simulink model "mission_server_leader_follower_qbot2_qbot2"  (Simulink 8.3)
settings: Solver=FixedStepDiscrete  StartTime=0.0  StopTime=inf  FixedStep=0.002  RelTol=1e-3
libraries: quarc_library x5, Orientation_Library x4
settings Model: Creator=glai  LastModifiedBy=user  SimulationMode=external  ExtModeTrigDuration=5000
settings SolverCC: PositivePriorityOrder=on
settings DataIOCC: SignalLoggingSaveFormat=Dataset
settings OptimizationCC: ExpressionDepthLimit=2147483647
settings RTWCC: SystemTargetFile=quarc_win64.tlc  TemplateMakefile=quarc_default_tmf  Description=QUARC Win64 Target  ProcessScript=quarc_win64_make_rtw_hook
settings STFCustomTargetCC: TargetPreCompLibLocation=C:\PROGRA~3\QUARC\lib\2014a\win64\release  CodeReplacementLibrary=C89/C90 (ANSI)  ConcurrentExecutionCompliant=on  GeneratePreprocessorConditionals=Disable all  CombineOutputUpdateFcns=on  CPPClassGenCompliant=on  GRTInterface=off  SystemTargetFile=quarc_win64.tlc
settings GRTTargetCC: TargetPreCompLibLocation=C:\PROGRA~3\QUARC\lib\2014a\win64\release  CodeReplacementLibrary=C89/C90 (ANSI)  ParMdlRefBuildCompliant=off  CompOptLevelCompliant=off  CombineOutputUpdateFcns=on  MatFileLogging=off  GRTInterface=off  ExtMode=on  ExtModeMexFile=quarc_comm  ExtModeMexArgs='-w -d %d -uri %u','shmem://%m:1?timeout=10'

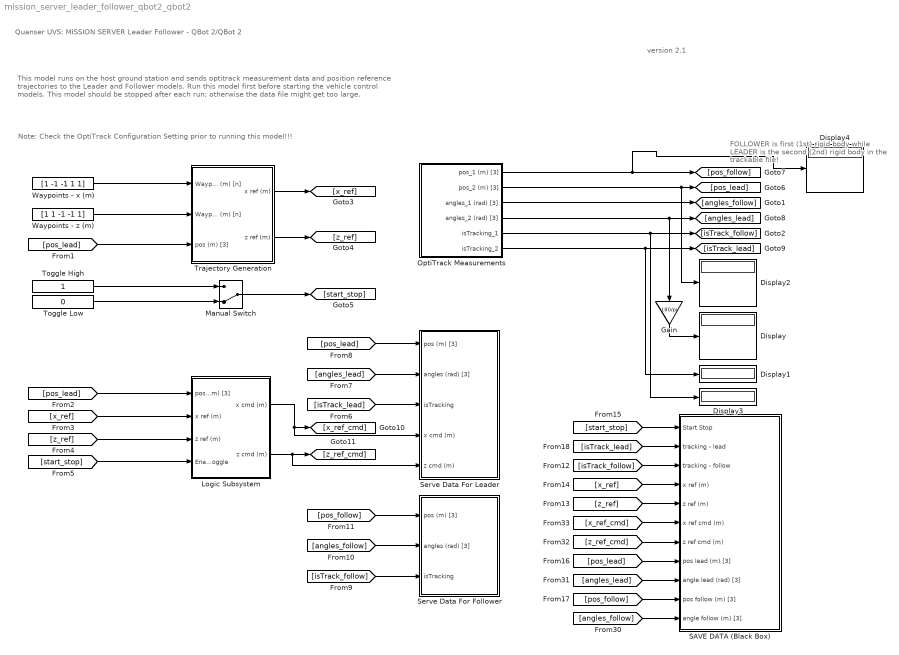
== system mission_server_leader_follower_qbot2_qbot2 ==
  note: FOLLOWER is first (1st) rigid body while
      | LEADER is the second (2nd) rigid body
      | in the trackable file!
  note: Note: Check the OptiTrack Configuration Setting prior to running this model!!!
  note: Quanser UVS: MISSION SERVER Leader Follower - QBot 2/QBot 2
  note: This model runs on the host ground station and sends
      | optitrack measurement data and position reference trajectories to the Leader and Follower models.
      | Run this model first before starting the vehicle control models.
      | This model should be stopped after each run; otherwise the data file might get too large.
  note: version 2.1
  Display{,1..4} (5 alike) : Display
      settings: Decimation=100
  Gain : Gain  Gain=180/pi
  Logic Subsystem : Subsystem
  Manual Switch : ManualSwitch  CurrentSetting=0
  OptiTrack Measurements : Subsystem
  SAVE DATA (Black Box) : Subsystem
  Serve Data For Follower : Subsystem
  Serve Data For Leader : Subsystem
  Toggle High : Constant
  Toggle Low : Constant  Value=0
  Trajectory Generation : Subsystem
  Waypoints - x (m) : Constant  Value=[1 -1 -1 1 1]
  Waypoints - z (m) : Constant  Value=[1 1 -1 -1 1]
  wires:
  Trajectory Generation/2(z ref (m)) -> [z_ref]
  Trajectory Generation/1(x ref (m)) -> [x_ref]
  [pos_lead] -> Logic Subsystem/1(pos (m) [3])
  [x_ref] -> Logic Subsystem/2(x ref (m))
  [start_stop] -> Logic Subsystem/4(Enable Toggle)
  [z_ref] -> Logic Subsystem/3(z ref (m))
  Logic Subsystem/1(x cmd (m)) -> [x_ref_cmd], Serve Data For Leader/4(x cmd (m))
  Logic Subsystem/2(z cmd (m)) -> [z_ref_cmd], Serve Data For Leader/5(z cmd (m))
  [angles_lead] -> Serve Data For Leader/2(angles (rad) [3])
  [isTrack_lead] -> Serve Data For Leader/3(isTracking)
  [pos_lead] -> Serve Data For Leader/1(pos (m) [3])
  Toggle High/1 -> Manual Switch/1
  Toggle Low/1 -> Manual Switch/2
  Manual Switch/1 -> [start_stop]
  Gain/1 -> Display/1
  OptiTrack Measurements/6(isTracking_2) -> Display1/1, [isTrack_lead]
  OptiTrack Measurements/5(isTracking_1) -> Display3/1, [isTrack_follow]
  OptiTrack Measurements/2(pos_2 (m) [3]) -> Display2/1, [pos_lead]
  OptiTrack Measurements/1(pos_1 (m) [3]) -> Display4/1, [pos_follow]
  OptiTrack Measurements/4(angles_2 (rad) [3]) -> Gain/1, [angles_lead]
  OptiTrack Measurements/3(angles_1 (rad) [3]) -> [angles_follow]
  [pos_follow] -> Serve Data For Follower/1(pos (m) [3])
  [angles_follow] -> Serve Data For Follower/2(angles (rad) [3])
  [isTrack_follow] -> Serve Data For Follower/3(isTracking)
  [z_ref] -> SAVE DATA (Black Box)/5(z ref (m))
  [start_stop] -> SAVE DATA (Black Box)/1(Start Stop)
  [x_ref] -> SAVE DATA (Black Box)/4(x ref (m))
  [pos_lead] -> SAVE DATA (Black Box)/8(pos lead (m) [3])
  [pos_follow] -> SAVE DATA (Black Box)/10(pos follow (m) [3])
  [angles_follow] -> SAVE DATA (Black Box)/11(angle follow (m) [3])
  [angles_lead] -> SAVE DATA (Black Box)/9(angle lead (rad) [3])
  [isTrack_follow] -> SAVE DATA (Black Box)/3(tracking - follow)
  [isTrack_lead] -> SAVE DATA (Black Box)/2(tracking - lead)
  [z_ref_cmd] -> SAVE DATA (Black Box)/7(z ref cmd (m))
  [x_ref_cmd] -> SAVE DATA (Black Box)/6(x ref cmd (m))
  Waypoints - z (m)/1 -> Trajectory Generation/2(Waypoint Z (m) [n])
  Waypoints - x (m)/1 -> Trajectory Generation/1(Waypoint X (m) [n])
  [pos_lead] -> Trajectory Generation/3(pos (m) [3])

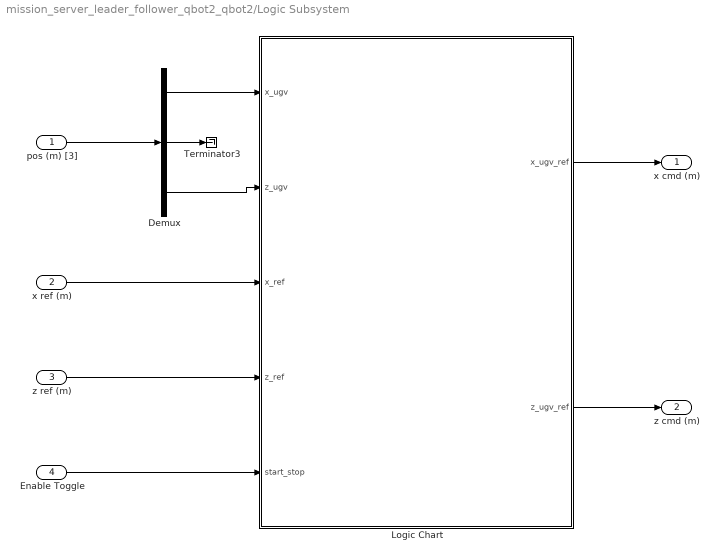
== system mission_server_leader_follower_qbot2_qbot2/Logic Subsystem ==
  pos (m) [3] : Inport
  x ref (m) : Inport  Port=2
  z ref (m) : Inport  Port=3
  Enable Toggle : Inport  Port=4
  Demux : Demux  Outputs=3
  Logic Chart : Stateflow chart  TreatAsAtomicUnit=on
  Terminator3 : Terminator
  x cmd (m) : Outport
  z cmd (m) : Outport  Port=2
  wires:
  pos (m) [3]/1 -> Demux/1
  Demux/2 -> Terminator3/1
  Demux/1 -> Logic Chart/1(x_ugv)
  Demux/3 -> Logic Chart/2(z_ugv)
  z ref (m)/1 -> Logic Chart/4(z_ref)
  Enable Toggle/1 -> Logic Chart/5(start_stop)
  x ref (m)/1 -> Logic Chart/3(x_ref)
  Logic Chart/1(x_ugv_ref) -> x cmd (m)/1
  Logic Chart/2(z_ugv_ref) -> z cmd (m)/1

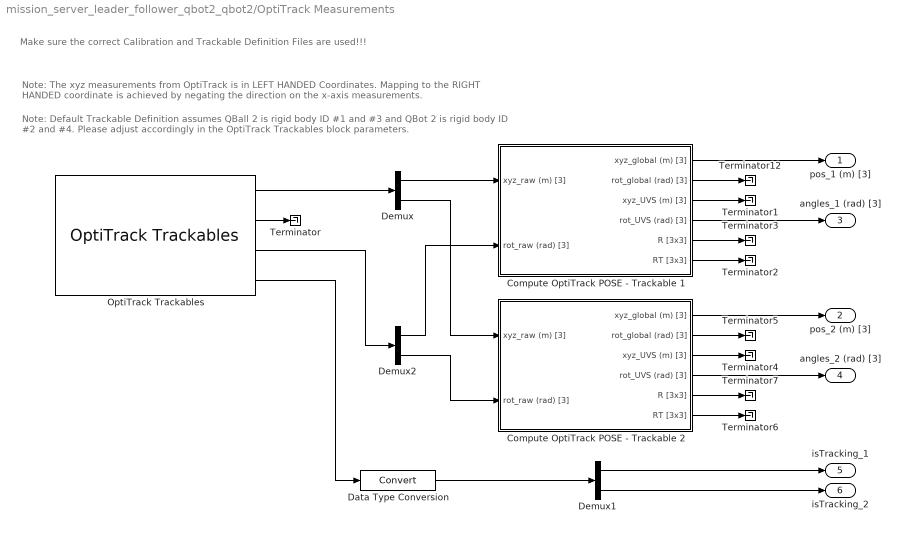
== system mission_server_leader_follower_qbot2_qbot2/OptiTrack Measurements ==
  note: Note: The xyz measurements from OptiTrack is in LEFT HANDED Coordinates.
      |
      | Mapping to the RIGHT HANDED coordinate is achieved by negating the direction on the x-axis measurements.
  note: Make sure the correct Calibration and Trackable Definition Files are used!!!
  note: Note: Default Trackable Definition assumes QBall 2 is rigid body ID #1 and #3 and QBot 2 is rigid body ID #2 and #4.
      | Please adjust accordingly in the OptiTrack Trackables block parameters.
  "Compute OptiTrack POSE - Trackable 1 " : Subsystem
  Compute OptiTrack POSE - Trackable 2 : Subsystem
  Data Type Conversion : DataTypeConversion
  Demux : Demux  Outputs=2
  Demux1 : Demux  Outputs=2
  Demux2 : Demux  Outputs=2
  OptiTrack Trackables : quarc_library/Devices/Third-Party/NaturalPoint/OptiTrack/OptiTrack Trackables  calibration_file=C:\Users\user\Desktop\final\Calibration Very High Quality Exceptional (MeanErr 0.001 mm) 2017-05-16 6.48pm.cal  rigid_body_file=C:\Users\user\Desktop\final\RigidBodies 2017-05-26 5.36pm_qbotx2.tra  rigid_body_ids=[1 2]  sample_time=qc_get_step_size
  Terminator{,1..7,12} (9 alike) : Terminator
  pos_1 (m) [3] : Outport
  pos_2 (m) [3] : Outport  Port=2
  angles_1 (rad) [3] : Outport  Port=3
  angles_2 (rad) [3] : Outport  Port=4
  isTracking_1 : Outport  Port=5
  isTracking_2 : Outport  Port=6
  wires:
  OptiTrack Trackables/1 -> Demux/1
  OptiTrack Trackables/2 -> Terminator/1
  OptiTrack Trackables/4 -> Data Type Conversion/1
  Data Type Conversion/1 -> Demux1/1
  Demux1/1 -> isTracking_1/1
  Demux1/2 -> isTracking_2/1
  OptiTrack Trackables/3 -> Demux2/1
  Demux/1 -> "Compute OptiTrack POSE - Trackable 1 "/1(xyz_raw (m) [3])
  Demux/2 -> Compute OptiTrack POSE - Trackable 2/1(xyz_raw (m) [3])
  Demux2/1 -> "Compute OptiTrack POSE - Trackable 1 "/2(rot_raw (rad) [3])
  Demux2/2 -> Compute OptiTrack POSE - Trackable 2/2(rot_raw (rad) [3])
  "Compute OptiTrack POSE - Trackable 1 "/1(xyz_global (m) [3]) -> pos_1 (m) [3]/1
  "Compute OptiTrack POSE - Trackable 1 "/2(rot_global (rad) [3]) -> Terminator12/1
  "Compute OptiTrack POSE - Trackable 1 "/3(xyz_UVS (m) [3]) -> Terminator1/1
  "Compute OptiTrack POSE - Trackable 1 "/4(rot_UVS (rad) [3]) -> angles_1 (rad) [3]/1
  "Compute OptiTrack POSE - Trackable 1 "/5(R [3x3]) -> Terminator3/1
  "Compute OptiTrack POSE - Trackable 1 "/6(RT [3x3]) -> Terminator2/1
  Compute OptiTrack POSE - Trackable 2/1(xyz_global (m) [3]) -> pos_2 (m) [3]/1
  Compute OptiTrack POSE - Trackable 2/2(rot_global (rad) [3]) -> Terminator5/1
  Compute OptiTrack POSE - Trackable 2/3(xyz_UVS (m) [3]) -> Terminator4/1
  Compute OptiTrack POSE - Trackable 2/4(rot_UVS (rad) [3]) -> angles_2 (rad) [3]/1
  Compute OptiTrack POSE - Trackable 2/5(R [3x3]) -> Terminator7/1
  Compute OptiTrack POSE - Trackable 2/6(RT [3x3]) -> Terminator6/1

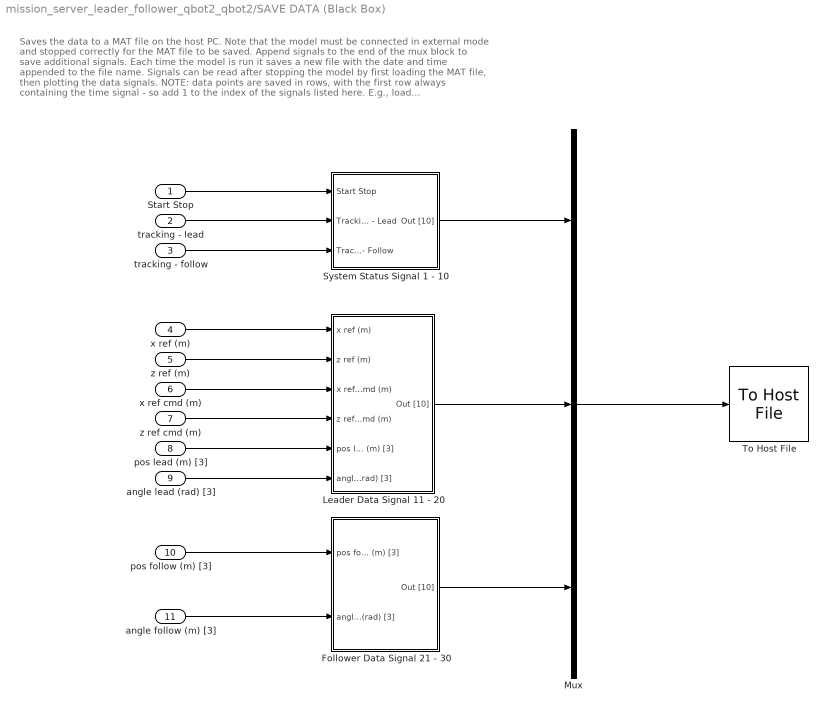
== system mission_server_leader_follower_qbot2_qbot2/SAVE DATA (Black Box) ==
  note: Saves the data to a MAT file on the host PC. Note that the model must be connected
      | in external mode and stopped correctly for the MAT file to be saved.
      | Append signals to the end of the mux block to save additional signals.
      | Each time the model is run it saves a new file with the date and time appended
      | to the file name.
      |
      | Signals can be read after stopping the model by first loading the MAT file, then plotting
      | the data signals. NOTE: data points are saved in rows, with the first row always containing
      | the time signal - so add 1 to the index of the signals listed here. E.g.,
      |
      | load mission_data.mat
      | t = mission_data(1,:);
      | roll = mission_data(22,:);
      | plot(t, roll);
  Start Stop : Inport
  tracking - lead : Inport  Port=2
  tracking - follow : Inport  Port=3
  x ref (m) : Inport  Port=4
  z ref (m) : Inport  Port=5
  x ref cmd (m) : Inport  Port=6
  z ref cmd (m) : Inport  Port=7
  pos lead (m) [3] : Inport  Port=8
  angle lead (rad) [3] : Inport  Port=9
  pos follow (m) [3] : Inport  Port=10
  angle follow (m) [3] : Inport  Port=11
  Follower Data Signal 21 - 30 : Subsystem
  Leader Data Signal 11 - 20 : Subsystem
  Mux : Mux  Inputs=3
  System Status Signal 1 - 10 : Subsystem
  To Host File : quarc_library/Sinks/To Host/To Host File  file_name=mission_data_%{date}_%{time}.mat  variable_name=mission_data  decimation=1  sample_time=-1  file_format=MAT-file v.4  options=No header or footer  append=off  final_file_name=mission_data_26-May-2017_18-02-36.mat
  wires:
  Start Stop/1 -> System Status Signal 1 - 10/1(Start Stop)
  tracking - follow/1 -> System Status Signal 1 - 10/3(Tracking - Follow)
  tracking - lead/1 -> System Status Signal 1 - 10/2(Tracking - Lead)
  z ref (m)/1 -> Leader Data Signal 11 - 20/2(z ref (m))
  x ref (m)/1 -> Leader Data Signal 11 - 20/1(x ref (m))
  pos lead (m) [3]/1 -> Leader Data Signal 11 - 20/5(pos lead (m) [3])
  angle lead (rad) [3]/1 -> Leader Data Signal 11 - 20/6(angle lead (rad) [3])
  System Status Signal 1 - 10/1(Out [10]) -> Mux/1
  Leader Data Signal 11 - 20/1(Out [10]) -> Mux/2
  Follower Data Signal 21 - 30/1(Out [10]) -> Mux/3
  pos follow (m) [3]/1 -> Follower Data Signal 21 - 30/1(pos follow (m) [3])
  angle follow (m) [3]/1 -> Follower Data Signal 21 - 30/2(angle follow (rad) [3])
  Mux/1 -> To Host File/1
  z ref cmd (m)/1 -> Leader Data Signal 11 - 20/4(z ref cmd (m))
  x ref cmd (m)/1 -> Leader Data Signal 11 - 20/3(x ref cmd (m))

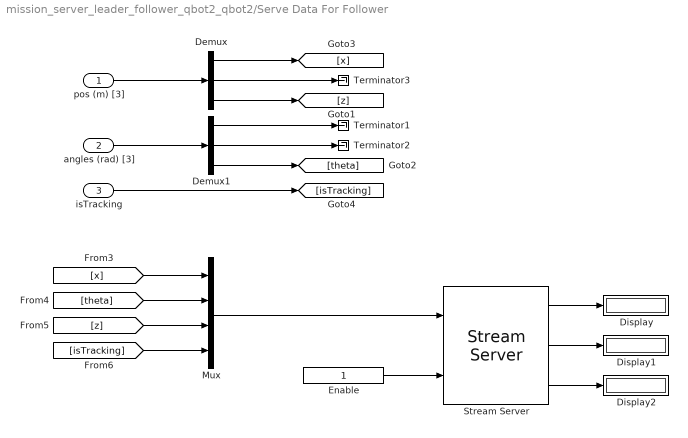
== system mission_server_leader_follower_qbot2_qbot2/Serve Data For Follower ==
  pos (m) [3] : Inport
  angles (rad) [3] : Inport  Port=2
  isTracking : Inport  Port=3
  Demux : Demux  Outputs=3
  Demux1 : Demux  Outputs=3
  Display : Display
      settings: Decimation=100
  Display1 : Display
      settings: Decimation=100
  Display2 : Display
      settings: Decimation=100
  Enable : Constant
  Mux : Mux
  Stream Server : quarc_library/Communications/Basic/Stream Server  uri_source=Specify via dialog (do not evaluate)  uri=tcpip://localhost:18005  apply_uri_to_all_configs=on  send_buffer_size=1460  receive_buffer_size=1460  byte_order=little endian (Intel - LSB first)  optimization=Minimum latency  implementation=Use non-blocking I/O  send_options=Send most recent data  receive_options=Do not receive data  send_fifo_size=1000  receive_fifo_size=1000  send_priority=0  receive_priority=0  default_value=[0]  send_dimensions=off  receive_dimensions=off  max_dimensions=-1  sample_time=qc_get_step_size  active=off  data_type=Inherited via back propagation  type_expr=BusObject
      settings: AttributesFormatString="\"tcpip://localhost:18005\""
  Terminator1 : Terminator
  Terminator2 : Terminator
  Terminator3 : Terminator
  wires:
  Stream Server/1 -> Display/1
  Stream Server/3 -> Display2/1
  Stream Server/2 -> Display1/1
  Mux/1 -> Stream Server/1
  Enable/1 -> Stream Server/2
  Demux1/1 -> Terminator1/1
  Demux1/2 -> Terminator2/1
  Demux1/3 -> [theta]
  isTracking/1 -> [isTracking]
  angles (rad) [3]/1 -> Demux1/1
  Demux/2 -> Terminator3/1
  Demux/1 -> [x]
  Demux/3 -> [z]
  pos (m) [3]/1 -> Demux/1
  [isTracking] -> Mux/4
  [z] -> Mux/3
  [theta] -> Mux/2
  [x] -> Mux/1

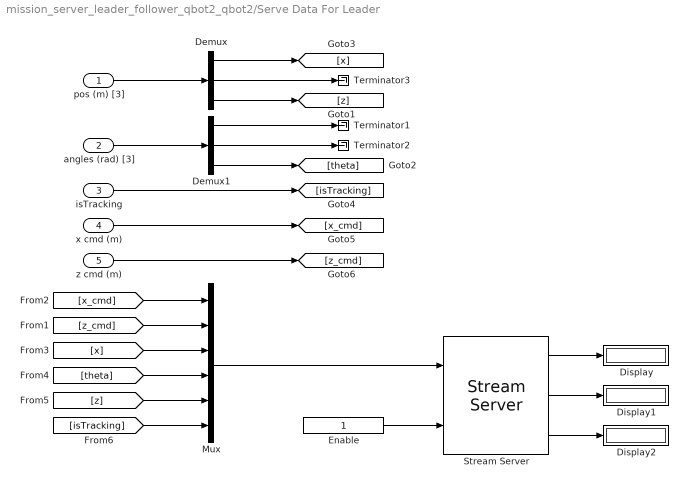
== system mission_server_leader_follower_qbot2_qbot2/Serve Data For Leader ==
  pos (m) [3] : Inport
  angles (rad) [3] : Inport  Port=2
  isTracking : Inport  Port=3
  x cmd (m) : Inport  Port=4
  z cmd (m) : Inport  Port=5
  Demux : Demux  Outputs=3
  Demux1 : Demux  Outputs=3
  Display : Display
      settings: Decimation=100
  Display1 : Display
      settings: Decimation=100
  Display2 : Display
      settings: Decimation=100
  Enable : Constant
  Mux : Mux  Inputs=6
  Stream Server : quarc_library/Communications/Basic/Stream Server  uri_source=Specify via dialog (do not evaluate)  uri=tcpip://localhost:18006  apply_uri_to_all_configs=on  send_buffer_size=1460  receive_buffer_size=1460  byte_order=little endian (Intel - LSB first)  optimization=Minimum latency  implementation=Use non-blocking I/O  send_options=Send most recent data  receive_options=Do not receive data  send_fifo_size=1000  receive_fifo_size=1000  send_priority=0  receive_priority=0  default_value=[0]  send_dimensions=off  receive_dimensions=off  max_dimensions=-1  sample_time=qc_get_step_size  active=off  data_type=Inherited via back propagation  type_expr=BusObject
      settings: AttributesFormatString="\"tcpip://localhost:18006\""
  Terminator1 : Terminator
  Terminator2 : Terminator
  Terminator3 : Terminator
  wires:
  pos (m) [3]/1 -> Demux/1
  Demux/3 -> [z]
  Demux/1 -> [x]
  Demux/2 -> Terminator3/1
  angles (rad) [3]/1 -> Demux1/1
  isTracking/1 -> [isTracking]
  Demux1/3 -> [theta]
  Demux1/2 -> Terminator2/1
  Demux1/1 -> Terminator1/1
  x cmd (m)/1 -> [x_cmd]
  z cmd (m)/1 -> [z_cmd]
  Enable/1 -> Stream Server/2
  Mux/1 -> Stream Server/1
  [x_cmd] -> Mux/1
  [theta] -> Mux/4
  [isTracking] -> Mux/6
  [z_cmd] -> Mux/2
  [z] -> Mux/5
  [x] -> Mux/3
  Stream Server/2 -> Display1/1
  Stream Server/3 -> Display2/1
  Stream Server/1 -> Display/1

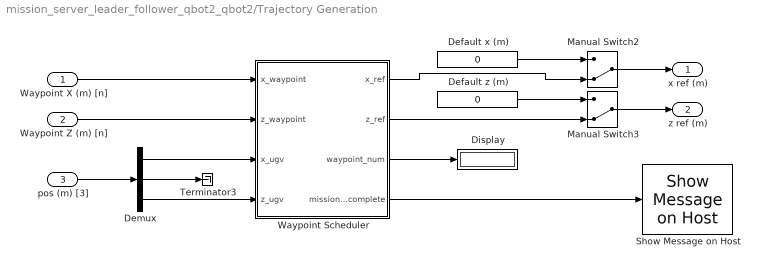
== system mission_server_leader_follower_qbot2_qbot2/Trajectory Generation ==
  Waypoint X (m) [n] : Inport
  Waypoint Z (m) [n] : Inport  Port=2
  pos (m) [3] : Inport  Port=3
  Default x (m) : Constant  Value=0
  Default z (m) : Constant  Value=0
  Demux : Demux  Outputs=3
  Display : Display
      settings: Decimation=100
  Manual Switch2 : ManualSwitch  CurrentSetting=0
  Manual Switch3 : ManualSwitch  CurrentSetting=0
  Show Message on Host : quarc_library/Sinks/Error Handling/Show Message on Host  message_type=Fixed error message  message_icon=Information  message=Final waypoint issued. Please stop all models when vehicle stops.
      settings: AttributesFormatString="\"%<message>\""
  Terminator3 : Terminator
  Waypoint Scheduler : MATLAB Function  TreatAsAtomicUnit=on
  x ref (m) : Outport
  z ref (m) : Outport  Port=2
  wires:
  Waypoint Scheduler/3(waypoint_num) -> Display/1
  Waypoint Scheduler/4(mission_complete) -> Show Message on Host/1
  Default x (m)/1 -> Manual Switch2/1
  Waypoint Scheduler/1(x_ref) -> Manual Switch2/2
  Default z (m)/1 -> Manual Switch3/1
  Waypoint Scheduler/2(z_ref) -> Manual Switch3/2
  Manual Switch2/1 -> x ref (m)/1
  Manual Switch3/1 -> z ref (m)/1
  Demux/1 -> Waypoint Scheduler/3(x_ugv)
  Demux/3 -> Waypoint Scheduler/4(z_ugv)
  pos (m) [3]/1 -> Demux/1
  Demux/2 -> Terminator3/1
  Waypoint X (m) [n]/1 -> Waypoint Scheduler/1(x_waypoint)
  Waypoint Z (m) [n]/1 -> Waypoint Scheduler/2(z_waypoint)

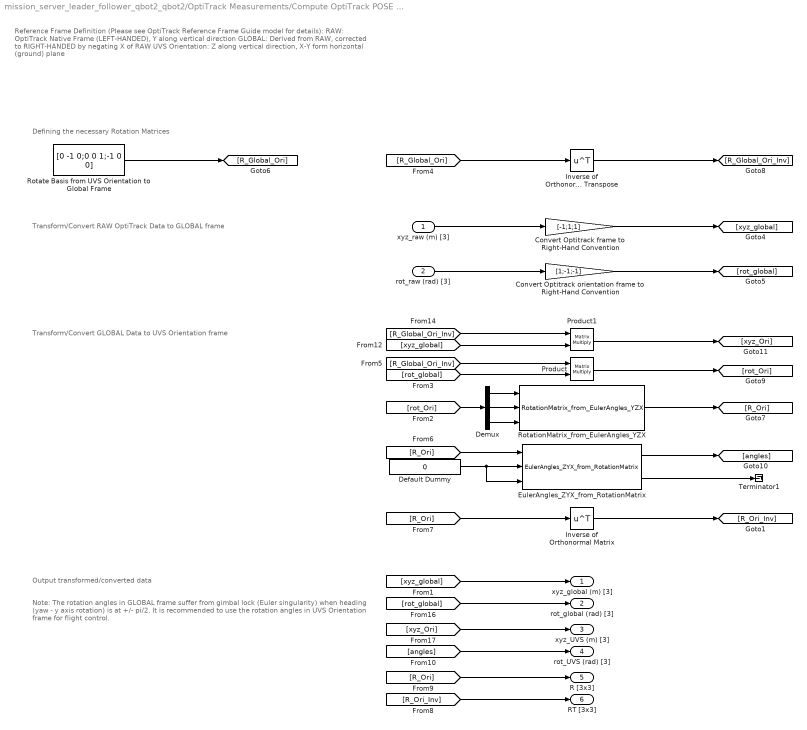
== system mission_server_leader_follower_qbot2_qbot2/OptiTrack Measurements/Compute OptiTrack POSE - Trackable 1  ==
  note: Transform/Convert RAW OptiTrack Data to GLOBAL frame
  note: Defining the necessary Rotation Matrices
  note: Reference Frame Definition (Please see OptiTrack Reference Frame Guide model for details):
      |
      | RAW: OptiTrack Native Frame (LEFT-HANDED), Y along vertical direction
      | GLOBAL: Derived from RAW, corrected to RIGHT-HANDED by negating X of RAW
      | UVS Orientation: Z along vertical direction, X-Y form horizontal (ground) plane
  note: Transform/Convert GLOBAL Data to UVS Orientation frame
  note: Output transformed/converted data
  note: Note: The rotation angles in GLOBAL frame suffer from gimbal lock (Euler singularity)
      | when heading (yaw - y axis rotation) is at +/- pi/2.
      | It is recommended to use the rotation angles in UVS Orientation frame for flight control.
  xyz_raw (m) [3] : Inport
  rot_raw (rad) [3] : Inport  Port=2
  Convert Optitrack frame to Right-Hand Convention : Gain  Gain=[-1;1;1]
  Convert Optitrack orientation frame to Right-Hand Convention : Gain  Gain=[1;-1;-1]
  Default Dummy : Constant  Value=0
  Demux : Demux  Outputs=3
  EulerAngles_ZYX_from_RotationMatrix : Orientation_Library/EulerAngles_ZYX_from_RotationMatrix
  Inverse of Orthonormal Matrix : Math  Operator=transpose  SaturateOnIntegerOverflow=on
  Inverse of Orthonormal Matrix is its Transpose : Math  Operator=transpose  SaturateOnIntegerOverflow=on
  Product : Product  Multiplication=Matrix(*)
  Product1 : Product  Multiplication=Matrix(*)
  Rotate Basis from UVS Orientation to Global Frame : Constant  Value=[0 -1 0;0 0 1;-1 0 0]
  RotationMatrix_from_EulerAngles_YZX : Orientation_Library/RotationMatrix_from_EulerAngles_YZX
  Terminator1 : Terminator
  xyz_global (m) [3] : Outport
  rot_global (rad) [3] : Outport  Port=2
  xyz_UVS (m) [3] : Outport  Port=3
  rot_UVS (rad) [3] : Outport  Port=4
  R [3x3] : Outport  Port=5
  RT [3x3] : Outport  Port=6
  wires:
  Rotate Basis from UVS Orientation to Global Frame/1 -> [R_Global_Ori]
  [R_Global_Ori] -> Inverse of Orthonormal Matrix is its Transpose/1
  Inverse of Orthonormal Matrix is its Transpose/1 -> [R_Global_Ori_Inv]
  Convert Optitrack orientation frame to Right-Hand Convention/1 -> [rot_global]
  xyz_raw (m) [3]/1 -> Convert Optitrack frame to Right-Hand Convention/1
  Convert Optitrack frame to Right-Hand Convention/1 -> [xyz_global]
  rot_raw (rad) [3]/1 -> Convert Optitrack orientation frame to Right-Hand Convention/1
  [R_Global_Ori_Inv] -> Product1/1
  [xyz_global] -> Product1/2
  Product1/1 -> [xyz_Ori]
  [R_Global_Ori_Inv] -> Product/1
  Product/1 -> [rot_Ori]
  [rot_global] -> Product/2
  [rot_Ori] -> Demux/1
  Demux/1 -> RotationMatrix_from_EulerAngles_YZX/1
  Demux/2 -> RotationMatrix_from_EulerAngles_YZX/2
  RotationMatrix_from_EulerAngles_YZX/1 -> [R_Ori]
  Demux/3 -> RotationMatrix_from_EulerAngles_YZX/3
  [R_Ori] -> EulerAngles_ZYX_from_RotationMatrix/1
  Default Dummy/1 -> EulerAngles_ZYX_from_RotationMatrix/3, EulerAngles_ZYX_from_RotationMatrix/2
  EulerAngles_ZYX_from_RotationMatrix/2 -> Terminator1/1
  EulerAngles_ZYX_from_RotationMatrix/1 -> [angles]
  [xyz_global] -> xyz_global (m) [3]/1
  [rot_global] -> rot_global (rad) [3]/1
  [xyz_Ori] -> xyz_UVS (m) [3]/1
  [angles] -> rot_UVS (rad) [3]/1
  [R_Ori] -> Inverse of Orthonormal Matrix/1
  Inverse of Orthonormal Matrix/1 -> [R_Ori_Inv]
  [R_Ori] -> R [3x3]/1
  [R_Ori_Inv] -> RT [3x3]/1

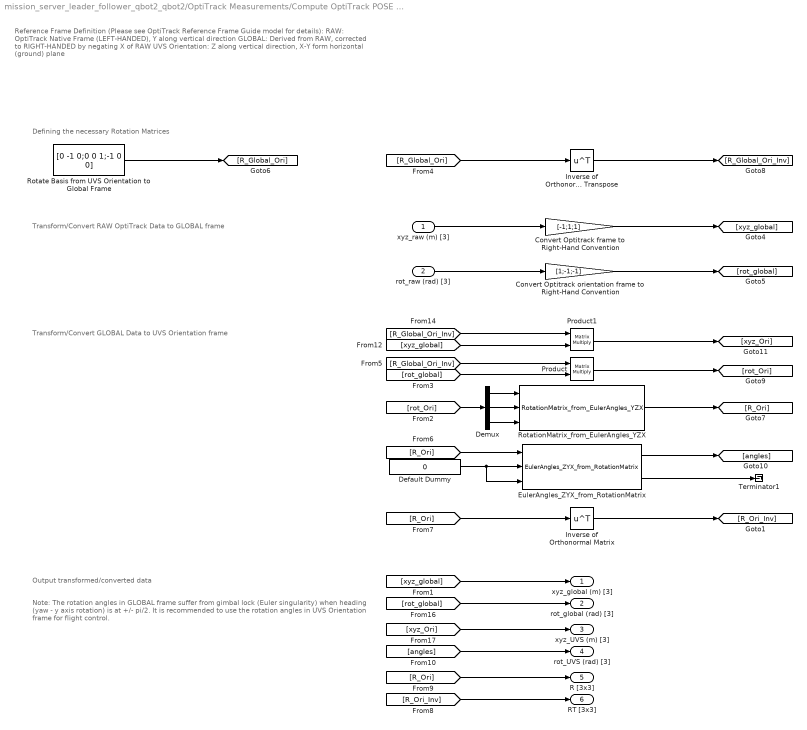
== system mission_server_leader_follower_qbot2_qbot2/OptiTrack Measurements/Compute OptiTrack POSE - Trackable 2 ==
  note: Note: The rotation angles in GLOBAL frame suffer from gimbal lock (Euler singularity)
      | when heading (yaw - y axis rotation) is at +/- pi/2.
      | It is recommended to use the rotation angles in UVS Orientation frame for flight control.
  note: Output transformed/converted data
  note: Transform/Convert GLOBAL Data to UVS Orientation frame
  note: Reference Frame Definition (Please see OptiTrack Reference Frame Guide model for details):
      |
      | RAW: OptiTrack Native Frame (LEFT-HANDED), Y along vertical direction
      | GLOBAL: Derived from RAW, corrected to RIGHT-HANDED by negating X of RAW
      | UVS Orientation: Z along vertical direction, X-Y form horizontal (ground) plane
  note: Defining the necessary Rotation Matrices
  note: Transform/Convert RAW OptiTrack Data to GLOBAL frame
  xyz_raw (m) [3] : Inport
  rot_raw (rad) [3] : Inport  Port=2
  Convert Optitrack frame to Right-Hand Convention : Gain  Gain=[-1;1;1]
  Convert Optitrack orientation frame to Right-Hand Convention : Gain  Gain=[1;-1;-1]
  Default Dummy : Constant  Value=0
  Demux : Demux  Outputs=3
  EulerAngles_ZYX_from_RotationMatrix : Orientation_Library/EulerAngles_ZYX_from_RotationMatrix
  Inverse of Orthonormal Matrix : Math  Operator=transpose  SaturateOnIntegerOverflow=on
  Inverse of Orthonormal Matrix is its Transpose : Math  Operator=transpose  SaturateOnIntegerOverflow=on
  Product : Product  Multiplication=Matrix(*)
  Product1 : Product  Multiplication=Matrix(*)
  Rotate Basis from UVS Orientation to Global Frame : Constant  Value=[0 -1 0;0 0 1;-1 0 0]
  RotationMatrix_from_EulerAngles_YZX : Orientation_Library/RotationMatrix_from_EulerAngles_YZX
  Terminator1 : Terminator
  xyz_global (m) [3] : Outport
  rot_global (rad) [3] : Outport  Port=2
  xyz_UVS (m) [3] : Outport  Port=3
  rot_UVS (rad) [3] : Outport  Port=4
  R [3x3] : Outport  Port=5
  RT [3x3] : Outport  Port=6
  wires:
  [R_Ori_Inv] -> RT [3x3]/1
  [R_Ori] -> R [3x3]/1
  Inverse of Orthonormal Matrix/1 -> [R_Ori_Inv]
  [R_Ori] -> Inverse of Orthonormal Matrix/1
  [angles] -> rot_UVS (rad) [3]/1
  [xyz_Ori] -> xyz_UVS (m) [3]/1
  [rot_global] -> rot_global (rad) [3]/1
  [xyz_global] -> xyz_global (m) [3]/1
  EulerAngles_ZYX_from_RotationMatrix/1 -> [angles]
  EulerAngles_ZYX_from_RotationMatrix/2 -> Terminator1/1
  Default Dummy/1 -> EulerAngles_ZYX_from_RotationMatrix/2, EulerAngles_ZYX_from_RotationMatrix/3
  [R_Ori] -> EulerAngles_ZYX_from_RotationMatrix/1
  Demux/3 -> RotationMatrix_from_EulerAngles_YZX/3
  RotationMatrix_from_EulerAngles_YZX/1 -> [R_Ori]
  Demux/2 -> RotationMatrix_from_EulerAngles_YZX/2
  Demux/1 -> RotationMatrix_from_EulerAngles_YZX/1
  [rot_Ori] -> Demux/1
  [rot_global] -> Product/2
  Product/1 -> [rot_Ori]
  [R_Global_Ori_Inv] -> Product/1
  Product1/1 -> [xyz_Ori]
  [xyz_global] -> Product1/2
  [R_Global_Ori_Inv] -> Product1/1
  rot_raw (rad) [3]/1 -> Convert Optitrack orientation frame to Right-Hand Convention/1
  Convert Optitrack frame to Right-Hand Convention/1 -> [xyz_global]
  xyz_raw (m) [3]/1 -> Convert Optitrack frame to Right-Hand Convention/1
  Convert Optitrack orientation frame to Right-Hand Convention/1 -> [rot_global]
  Inverse of Orthonormal Matrix is its Transpose/1 -> [R_Global_Ori_Inv]
  [R_Global_Ori] -> Inverse of Orthonormal Matrix is its Transpose/1
  Rotate Basis from UVS Orientation to Global Frame/1 -> [R_Global_Ori]

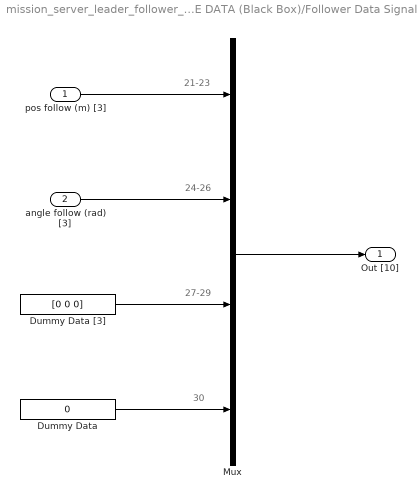
== system mission_server_leader_follower_qbot2_qbot2/SAVE DATA (Black Box)/Follower Data Signal 21 - 30 ==
  note: 30
  note: 27-29
  note: 24-26
  note: 21-23
  pos follow (m) [3] : Inport
  angle follow (rad) [3] : Inport  Port=2
  Dummy Data : Constant  Value=0
  Dummy Data [3] : Constant  Value=[0 0 0]
  Mux : Mux  Inputs=[3 3 3 1]
  Out [10] : Outport
  wires:
  Mux/1 -> Out [10]/1
  pos follow (m) [3]/1 -> Mux/1
  angle follow (rad) [3]/1 -> Mux/2
  Dummy Data [3]/1 -> Mux/3
  Dummy Data/1 -> Mux/4

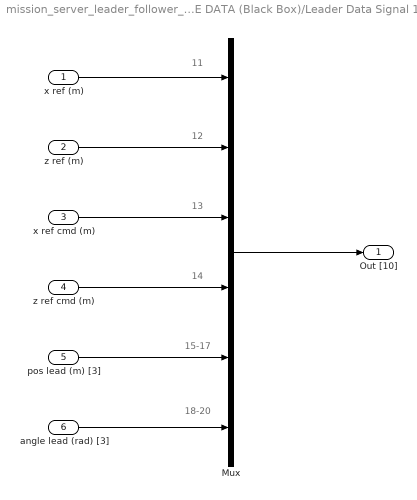
== system mission_server_leader_follower_qbot2_qbot2/SAVE DATA (Black Box)/Leader Data Signal 11 - 20 ==
  note: 11
  note: 12
  note: 13
  note: 15-17
  note: 14
  note: 18-20
  x ref (m) : Inport
  z ref (m) : Inport  Port=2
  x ref cmd (m) : Inport  Port=3
  z ref cmd (m) : Inport  Port=4
  pos lead (m) [3] : Inport  Port=5
  angle lead (rad) [3] : Inport  Port=6
  Mux : Mux  Inputs=[1 1 1 1 3 3]
  Out [10] : Outport
  wires:
  Mux/1 -> Out [10]/1
  x ref (m)/1 -> Mux/1
  z ref (m)/1 -> Mux/2
  x ref cmd (m)/1 -> Mux/3
  z ref cmd (m)/1 -> Mux/4
  pos lead (m) [3]/1 -> Mux/5
  angle lead (rad) [3]/1 -> Mux/6

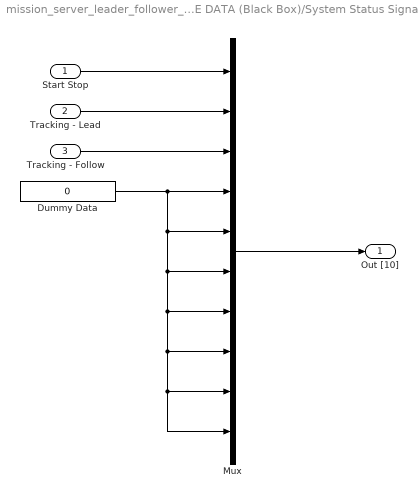
== system mission_server_leader_follower_qbot2_qbot2/SAVE DATA (Black Box)/System Status Signal 1 - 10 ==
  Start Stop : Inport
  Tracking - Lead : Inport  Port=2
  Tracking - Follow : Inport  Port=3
  Dummy Data : Constant  Value=0
  Mux : Mux  Inputs=10
  Out [10] : Outport
  wires:
  Tracking - Follow/1 -> Mux/3
  Tracking - Lead/1 -> Mux/2
  Start Stop/1 -> Mux/1
  Dummy Data/1 -> Mux/7, Mux/8, Mux/9, Mux/10, Mux/6, Mux/5, Mux/4
  Mux/1 -> Out [10]/1

== matlab function Trajectory Generation/Waypoint Scheduler ==
  data: x_waypoint input double; x_ref output double; z_waypoint input double; x_ugv input double; z_ugv input double; z_ref output double; waypoint_num output double; mission_complete output double
function [x_ref, z_ref, waypoint_num, mission_complete] = fcn(x_waypoint, z_waypoint, x_ugv, z_ugv)
%#codegen

% This function generates a trajectory to be tracked based on a vector of
% waypoint positions that get passed in. We increment the
% index into the waypoint vector once the vehicle has got to within a
% pre-determined threshold of the waypoint. 

persistent idx

if isempty(idx)
    idx = 1;
end

mission_complete = 0;

% The distance below which we switch to the next waypoint:
DIST_THRESHOLD = 0.15;

% Check if we're still far enough away from the waypoint:
dist = norm([x_ugv - x_waypoint(idx), z_ugv - z_waypoint(idx)], 2);

if dist > DIST_THRESHOLD || idx == length(x_waypoint)
    x_ref = x_waypoint(idx);
    z_ref = z_waypoint(idx);
else % Move to the next waypoint
    idx = idx + 1;
    x_ref = x_waypoint(idx);
    z_ref = z_waypoint(idx);
end

waypoint_num = idx;

% Check if the mission is finished:
if idx == length(x_waypoint)
    mission_complete = 1;
end

== stateflow chart Logic Subsystem/Logic Chart ==
  state WaitForStartCommand
    du:
    x_ugv_ref = x_ugv
    z_ugv_ref = z_ugv
  state QbotGetsWaypoints
    du:
    x_ugv_ref = x_ref
    z_ugv_ref = z_ref
  (default) -> WaitForStartCommand
  QbotGetsWaypoints -> WaitForStartCommand : [hasChanged(start_stop)]
  WaitForStartCommand -> QbotGetsWaypoints : [hasChanged(start_stop)]
  data: x_ugv input double; z_ugv input double; x_ref input double; z_ref input double; x_ugv_ref output double; z_ugv_ref output double; start_stop input double
